simulink model "progetto1_0"  (R2020b)
settings: Solver=VariableStepAuto  StartTime=0.0  StopTime=6  RelTol=1e-3
undefined symbols (not defined in the file): DiscIntNeverNeededParam, duration, force_type, fx, fy, fz, link, link_name, model_name, quadrotor, torque_type, tx, ty, tz
libraries: robotgazebolib x7, simulink x6
settings Model: Creator=mosca  LastModifiedBy=mosca

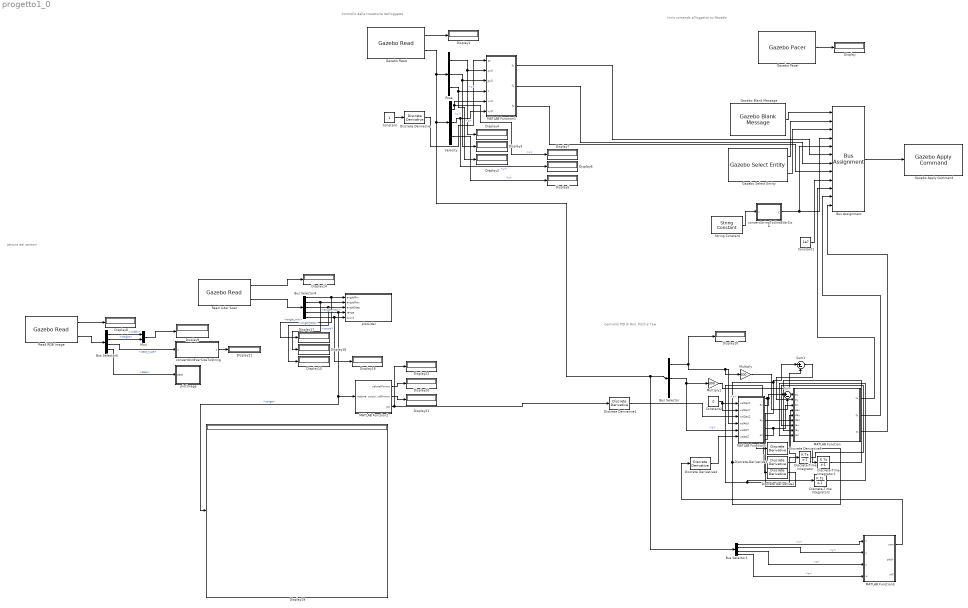
== system progetto1_0 ==
  note: Invio comando all'oggetto su Gazebo
  note: Controllo PID di Roll, Pitch e Yaw
  note: Controllo della traiettoria dell'oggetto
  note: Lettura dei sensori
  Bus Assignment : BusAssignment  AssignedSignals=model_name,link_name,force_type,torque_type,fx,fy,fz,duration.nano_seconds,tx,ty,tz
  Bus Selector : BusSelector  OutputSignals=world_angular_velocity.x,world_angular_velocity.y,world_angular_velocity.z
  Bus Selector1 : BusSelector  OutputSignals=world_pose.orientation.x,world_pose.orientation.y,world_pose.orientation.z,world_pose.orientation.w
  Bus Selector4 : BusSelector  OutputSignals=angle_min,angle_max,angle_step,range,count
  Bus Selector5 : BusSelector  OutputSignals=width,height,data_type,data
  Constant : Constant
  Constant1 : Constant  Value=1e7
  Constant2 : Constant  Value=0
  Discrete Derivative{,1..4,6} (6 alike) : simulink/Discrete/Discrete Derivative  gainval=1.0  ICPrevScaledInput=0.0  OutMin=[]  OutMax=[]  OutDataType=fixdt(1, 16)  OutScaling=2^-10  DoSatur=off
  Discrete-Time Integrator : DiscreteIntegrator  SampleTime=-1  ICPrevOutput=DiscIntNeverNeededParam  ICPrevScaledInput=DiscIntNeverNeededParam
  Discrete-Time Integrator1 : DiscreteIntegrator  SampleTime=-1  ICPrevOutput=DiscIntNeverNeededParam  ICPrevScaledInput=DiscIntNeverNeededParam
  Discrete-Time Integrator2 : DiscreteIntegrator  SampleTime=-1  ICPrevOutput=DiscIntNeverNeededParam  ICPrevScaledInput=DiscIntNeverNeededParam
  Display{,1..11,14..22} (21 alike) : Display
  Gazebo Apply Command : robotgazebolib/Gazebo Apply Command  cmdType=ApplyLinkWrench  sampleTime=0.001
      settings: SourceProductBaseCode=RO
  Gazebo Blank Message : robotgazebolib/Gazebo Blank Message  msgType=ApplyLinkWrench  sampleTime=0.001  busName='Gazebo_SL_Bus_gazebo_msgs_ApplyLinkWrench'
      settings: SourceProductBaseCode=RO
  Gazebo Pacer : robotgazebolib/Gazebo Pacer  ResetBehavior=Reset Gazebo simulation time and scene  SampleTime=0.001
      settings: SourceProductBaseCode=RO
  Gazebo Read : robotgazebolib/Gazebo Read  topicSource=From Gazebo  topic=/gazebo/ground_truth/link_state/quadrotor/link  messageType=gazebo_msgs/LinkState  sampleTime=0.001
      settings: SourceProductBaseCode=RO
  Gazebo Select Entity : robotgazebolib/Gazebo Select Entity  modelElemName=quadrotor/link  outputArraySize=128  OutputLabel=Link  SelectType=Link
      settings: SourceProductBaseCode=RO
  MATLAB Function : MATLAB Function  TreatAsAtomicUnit=on
  MATLAB Function1 : MATLAB Function  TreatAsAtomicUnit=on
  MATLAB Function2 : MATLAB Function  TreatAsAtomicUnit=on
  MATLAB Function3 : MATLAB Function  TreatAsAtomicUnit=on
  MATLAB Function5 : MATLAB Function  TreatAsAtomicUnit=on
  Multiply : Gain  Gain=200
  Multiply1 : Gain  Gain=300
  Mux : Mux  Inputs=2
  Pose : BusSelector  OutputSignals=world_pose.position.x,world_pose.position.y,world_pose.position.z
  Read Lidar Scan : robotgazebolib/Gazebo Read  topicSource=From Gazebo  topic=/gazebo/default/quadrotor/hokuyo/link/laser/scan  messageType=gazebo_msgs/LaserScan  sampleTime=0.001
      settings: SourceProductName=Robotics System Toolbox
  Read RGB Image : robotgazebolib/Gazebo Read  topicSource=From Gazebo  topic=/gazebo/default/quadrotor/camera/link/camera/image  messageType=gazebo_msgs/Image  sampleTime=0.001
      settings: SourceProductName=Robotics System Toolbox
  String Constant : StringConstant  String="\"SET\""
  Sum : Sum  Inputs=|+-
  Sum1 : Sum  Inputs=|+-
  Velocity : BusSelector  OutputSignals=world_linear_velocity.x,world_linear_velocity.y,world_linear_velocity.z
  convertStringToUInt8VarSize : MATLAB Function  TreatAsAtomicUnit=on
  convertUIn8VarSizeToString : MATLAB Function  TreatAsAtomicUnit=on
  plotImage : MATLAB Function  TreatAsAtomicUnit=on
  plotLidar : MATLAB Function  TreatAsAtomicUnit=on
  wires:
  Gazebo Pacer/1 -> Display/1
  Gazebo Blank Message/1 -> Bus Assignment/1
  Gazebo Read/1 -> Display1/1
  Pose/3 -> Display2/1, MATLAB Function1/4(z)  "<z>"
  Pose/1 -> Display4/1, MATLAB Function1/2(px0)  "<x>"
  Pose/2 -> Display3/1, MATLAB Function1/3(py0)  "<y>"
  Constant/1 -> Discrete Derivative/1
  Discrete Derivative/1 -> MATLAB Function1/1(az)
  MATLAB Function1/1(fx) -> Bus Assignment/6
  MATLAB Function1/2(fy) -> Bus Assignment/7
  MATLAB Function1/3(fz) -> Bus Assignment/8
  Constant1/1 -> Bus Assignment/9
  Gazebo Select Entity/1 -> Bus Assignment/2
  Gazebo Select Entity/2 -> Bus Assignment/3
  String Constant/1 -> convertStringToUInt8VarSize/1(u)
  convertStringToUInt8VarSize/1(y) -> Bus Assignment/4, Bus Assignment/5
  Bus Assignment/1 -> Gazebo Apply Command/1
  Velocity/1 -> Display7/1, MATLAB Function1/5(vx0)  "<x>"
  Velocity/2 -> Display6/1, MATLAB Function1/6(vy0)  "<y>"
  Velocity/3 -> Display5/1  "<z>"
  Read Lidar Scan/1 -> Display14/1
  Read Lidar Scan/2 -> Bus Selector4/1
  Bus Selector4/3 -> Display15/1, plotLidar/3(angleStep)  "<angle_step>"
  Bus Selector4/5 -> Display18/1, plotLidar/5(count)  "<count>"
  Bus Selector4/4 -> Display19/1, MATLAB Function2/1(vettore), plotLidar/4(range)  "<range>"
  Bus Selector4/1 -> Display17/1, plotLidar/1(angleMin)  "<angle_min>"
  Bus Selector4/2 -> Display16/1, plotLidar/2(angleMax)  "<angle_max>"
  MATLAB Function2/1(valoreMinimo) -> Display20/1
  MATLAB Function2/2(posizioneMinimo) -> Display21/1
  convertUIn8VarSizeToString/1(y) -> Display11/1
  Bus Selector5/4 -> plotImage/1(data)  "<data>"
  Bus Selector5/2 -> Mux/2  "<height>"
  Mux/1 -> Display9/1
  Read RGB Image/2 -> Bus Selector5/1
  Bus Selector5/1 -> Mux/1  "<width>"
  Read RGB Image/1 -> Display8/1
  Bus Selector5/3 -> convertUIn8VarSizeToString/1(u)  "<data_type>"
  MATLAB Function/1(tx) -> Bus Assignment/10
  MATLAB Function/2(ty) -> Bus Assignment/11
  MATLAB Function/3(tz) -> Bus Assignment/12
  Multiply1/1 -> Sum1/2
  Bus Selector1/1 -> MATLAB Function3/1(x)  "<x>"
  MATLAB Function3/1(yaw) -> Discrete Derivative4/1
  Sum1/1 -> MATLAB Function/2(ey)
  Bus Selector1/2 -> MATLAB Function3/2(y)  "<y>"
  Bus Selector1/4 -> MATLAB Function3/4(w)  "<w>"
  Multiply/1 -> Sum/2
  Discrete-Time Integrator2/1 -> MATLAB Function/9(iez)
  Discrete-Time Integrator/1 -> MATLAB Function/7(iex)
  Gazebo Read/2 -> Bus Selector1/1, Bus Selector/1, Velocity/1, Pose/1
  MATLAB Function5/3(ez) -> Discrete Derivative2/1, MATLAB Function/3(ez)
  Constant2/1 -> MATLAB Function5/2(velDesY), MATLAB Function5/1(velDesX)
  Discrete Derivative3/1 -> MATLAB Function/5(dey)
  Discrete Derivative6/1 -> MATLAB Function/4(dex)
  Discrete-Time Integrator1/1 -> MATLAB Function/8(iey)
  MATLAB Function2/3(psi) -> Discrete Derivative1/1, Display22/1
  Bus Selector1/3 -> MATLAB Function3/3(z)  "<z>"
  Discrete Derivative2/1 -> MATLAB Function/6(dez)
  Bus Selector/2 -> Multiply1/1, MATLAB Function5/5(velAttY)  "<y>"
  Discrete Derivative4/1 -> MATLAB Function5/6(velAttZ)
  MATLAB Function5/2(ey) -> Sum1/1, Discrete-Time Integrator1/1, Discrete Derivative3/1
  Sum/1 -> MATLAB Function/1(ex)
  Bus Selector/1 -> Multiply/1, MATLAB Function5/4(velAttX), Display10/1  "<x>"
  MATLAB Function5/1(ex) -> Sum/1, Discrete-Time Integrator2/1, Discrete-Time Integrator/1, Discrete Derivative6/1
  Discrete Derivative1/1 -> MATLAB Function5/3(velDesZ)

== matlab function progetto1_0/plotImage ==
  data: data input
function plotImage(data)

coder.extrinsic('imshow');
coder.extrinsic('helperPlotImage');

persistent h

if isempty(h)
    h = newplot(figure());
end


y = zeros(240, 320, 3, 'uint8');
if ~isempty(data) && ~isscalar(data)
    y(:) = helperPlotImage(data);
end
imshow(y, 'Parent', h);

== matlab function progetto1_0/MATLAB Function1 ==
  data: az input; fx output; px0 input; py0 input; z input; fy output; fz output; vx0 input; vy0 input
function [fx, fy, fz] = fcn(az , px0, py0, z, vx0, vy0)

t = 0.2;
m = 1.32+0.1+0.1;
px = 5*cos(z);
py = 5*sin(z);

ax = (2*(px - (vx0*t) - px0))/(t^2);
ay =(2*(py - (vy0*t) - py0))/(t^2);

% ax = (2*(px  - px0))/(t^2);
% ay = (2*(py  - py0))/(t^2);


fx = ax*m;
fy = ay*m;
fz = m*(9.8+az);

== matlab function progetto1_0/plotLidar ==
  data: angleMin input; angleMax input; angleStep input; range input; count input
function plotLidar(angleMin, angleMax, angleStep, range, count)

%plotLidar plot Lidar Scans
coder.extrinsic('lidarScan');
coder.extrinsic('plot');

persistent h

if isempty(h)
    h = newplot(figure());
end

if count ~= 0
    plot(lidarScan(range, angleMin:angleStep:angleMax), 'Parent', h);
    grid(h, 'on');
    axis(h, 'equal');
    view(h, -90, 90);
    xlabel(h, 'X');
    ylabel(h, 'Y');
end

end

== matlab function progetto1_0/MATLAB Function2 ==
  data: vettore input; valoreMinimo output; posizioneMinimo output; psi output
function [valoreMinimo, posizioneMinimo, psi] = fnc(vettore)
%funzione per trovare la posizione dell'elemtento del LIDAR più vicino
%all'oggetto
valoreMinimo = Inf;
posizioneMinimo = 0;

% Iterazione attraverso il vettore
    for i = 1:length(vettore)
     % Controllo se l'elemento è diverso da zero e minore del valore minimo attuale
        if vettore(i) ~= 0 && vettore(i) < valoreMinimo
            valoreMinimo = vettore(i);  % Aggiornamento del valore minimo
            posizioneMinimo = i;        % Aggiornamento della posizione del valore minimo
        end
    end

psi = (((2*pi)/640)*posizioneMinimo);

== matlab function progetto1_0/convertStringToUInt8VarSize ==
  data: u input; y output size=128
function y = convertStringToUInt8VarSize(u)

y = uint8(convertStringsToChars(u))';

== matlab function progetto1_0/MATLAB Function3 ==
  data: x input; yaw output; y input; z input; w input; pitch output; roll output
function  [yaw, pitch, roll] = fcn(x, y, z, w)
%trasforma quaternioni in angoli di eulero
quat=[x,y,z,w];
u = quat2eul(quat);

yaw = abs(u(1));
pitch = u(2);
roll = u(3);

== matlab function progetto1_0/MATLAB Function ==
  data: ex input; tx output; ey input; ez input; dex input; dey input; dez input; iex input; iey input; iez input; ty output; tz output
function [tx, ty, tz] = control(ex, ey, ez, dex, dey, dez, iex, iey, iez)

kp = 1;
kd = 0;
ki = 0;
tx = 5*(ex) + (kd*dex) + (ki*iex);
ty = 5*(ey) + (kd*dey) + (ki*iey);
tz = 20*(ez) + (kd*dez) + (ki*iez) ;

== matlab function progetto1_0/convertUIn8VarSizeToString ==
  data: u input; y output string
function y = convertUInt8VarSizeToString(u)

y = convertCharsToStrings(char(u'));

== matlab function progetto1_0/MATLAB Function5 ==
  data: velDesX input; ex output; velDesY input; velDesZ input; velAttX input; velAttY input; velAttZ input; ey output; ez output
function [ex, ey, ez] = fcn(velDesX, velDesY, velDesZ, velAttX, velAttY, velAttZ)

ex = velDesX - velAttX;
ey = velDesY - velAttY;
ez = velDesZ - velAttZ;
